simulink model "vector"  (R2025a)
settings: Solver=VariableStepAuto  StartTime=0.0  StopTime=5  RelTol=1e-3
libraries: spsCurrentMeasurementLib x3, spsVoltageMeasurementLib x2, spsAsynchronousMachineSIUnitsLib x1, spsDCVoltageSourceLib x1, eeHysteresisControl x1, spsUniversalBridgeLib x1, sps_lib x1
settings Model: Creator=aditl  LastModifiedBy=aditl

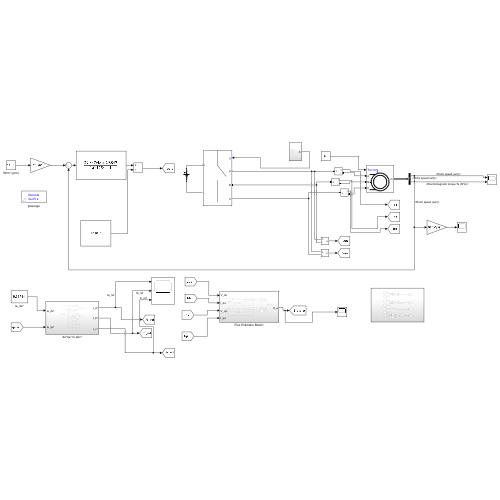
[thumbnail: Simulink's stored preview of the top-level diagram]
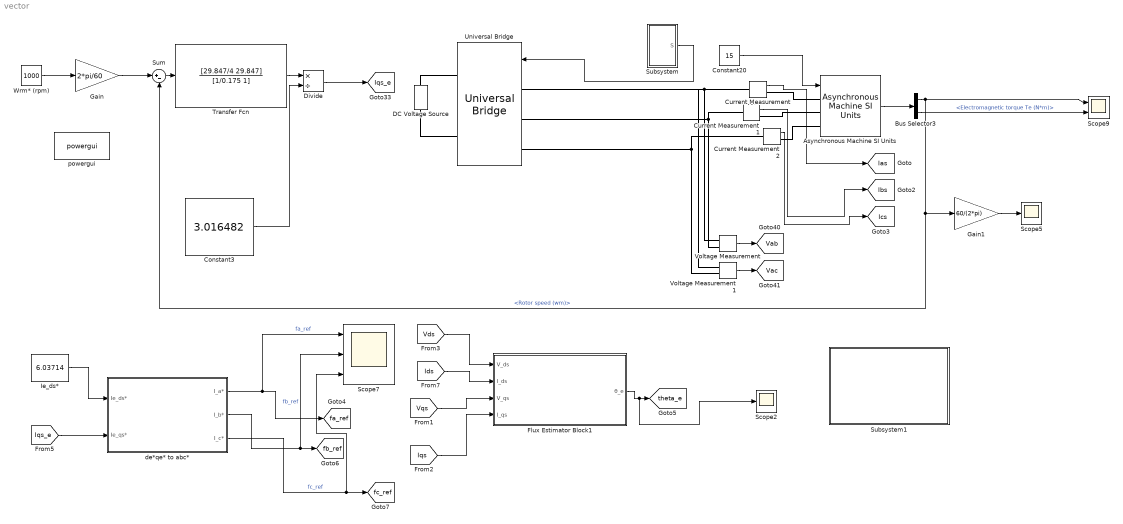
== system vector ==
  Asynchronous Machine SI Units : spsAsynchronousMachineSIUnitsLib/Asynchronous Machine SI Units  RotorType=Squirrel-cage  PresetModel="15:  5.4 HP (4KW)   400 V  50Hz 1430 RPM"  MechanicalLoad=Torque Tm  ShowDetailedParameters=on  ReferenceFrame=Stationary  Units=SI  MeasurementBus=off  NominalParameters=[4000 400 50]  VoltageRatio=1  Stator=[1.405 0.005839]  Rotor=[1.395 0.005839]  Cage1=[0.4155 0.002066]  Cage2=[0.4168 0.0003495]  Lm=0.1722  Mechanical=[0.0131 0.002985 2]  PolePairs=2  InitialConditions=[0 10 0 0 0 0 0 0]  SimulateSaturation=off  Saturation=[14.03593122, 27.81365428, 53.79336849, 72.68890987, 97.98006896, 148.6815601, 215.7428561, 302.9841135, 428.7778367 ; 230, 322, 414, 460, 506, 552, 598, 644, 690]  LoadFlowParameters=1492000  TsPowergui=0  TsBlock=-1  IterativeModel=Trapezoidal non iterative  IterativeDiscreteModel=Trapezoidal non iterative  Pmec=1.492e+006
  Bus Selector3 : BusSelector  OutputSignals=Mechanical.Rotor speed (wm),Mechanical.Electromagnetic torque Te (N*m)
  Constant20 : Constant  Value=15
  Constant3 : Constant  Value=3.016482
  Current Measurement : spsCurrentMeasurementLib/Current Measurement  PhasorSimulation=off  OutputType=Complex  PSBequivalent=0
  Current Measurement1 : spsCurrentMeasurementLib/Current Measurement  PhasorSimulation=off  OutputType=Complex  PSBequivalent=0
  Current Measurement2 : spsCurrentMeasurementLib/Current Measurement  PhasorSimulation=off  OutputType=Complex  PSBequivalent=0
  DC Voltage Source : spsDCVoltageSourceLib/DC Voltage Source  Amplitude=1088.662  Measurements=None
  Divide : Product  Inputs=*/
  Flux Estimator Block1 : Subsystem
  Gain : Gain  Gain=2*pi/60
  Gain1 : Gain  Gain=60/(2*pi)
  Ie_ds* : Constant  Value=6.03714
  Scope2 : Scope
      settings: ActiveDisplayYMinimum=-3.926985235827948  ActiveDisplayYMaximum=3.9269805856564539
  Scope5 : Scope
      settings: ActiveDisplayYMinimum=-1164.848987364373  ActiveDisplayYMaximum=1796.0943319293749  DataLoggingVariableName=ScopeData5
  Scope7 : Scope  NumInputPorts=3
      settings: ActiveDisplayYMinimum=-753403.64622958587  ActiveDisplayYMaximum=359759.36964912462  DataLoggingVariableName=ScopeData7
  Scope9 : Scope  NumInputPorts=2
      settings: ActiveDisplayYMinimum=45.4669289684437  ActiveDisplayYMaximum=169.48104420293922  DataLoggingVariableName=ScopeData9
  Subsystem : Subsystem
  Subsystem1 : Subsystem
  Sum : Sum  Inputs=|+-
  Transfer Fcn : TransferFcn  Numerator=[29.847/4 29.847]  Denominator=[1/0.175 1]
  Universal Bridge : spsUniversalBridgeLib/Universal Bridge  Arms=3  SnubberResistance=1e5  SnubberCapacitance=inf  Device=Ideal Switches  Ron=1e-3  Lon=0  ForwardVoltages="[  0  0  ]"  ForwardVoltage=0  GTOparameters=[ 10e-6 , 20e-6 ]  IGBTparameters=[ 1e-6 , 2e-6 ]  Measurements=None  Measurements_2=None  converterType=Rectifier
  Voltage Measurement : spsVoltageMeasurementLib/Voltage Measurement  PhasorSimulation=off  OutputType=Complex  PSBequivalent=0
  Voltage Measurement1 : spsVoltageMeasurementLib/Voltage Measurement  PhasorSimulation=off  OutputType=Complex  PSBequivalent=0
  Wrm* (rpm) : Constant  Value=1000
  de*qe* to abc* : Subsystem
  powergui : sps_lib/powergui  Priority=1  SimulationMode=Discrete  SampleTime=50e-6  frequency=60  Iterations=50  frequencyindice=50  Pbase=100e6  ErrMax=1e-4  UnitsV=kV  UnitsW=MW  buscounter=0  FunctionMessages=off  echomessages=off  EnableUseOfTLC=off  CurrentSourceSwitches=off  DisableSnubberDevices=off  DisableRonSwitches=off  DisableVfSwitches=off  DisplayEquations=off  AutomaticDiscreteSolvers=off  SolverType=Tustin/Backward Euler (TBE)  Interpol=off  ExternalGateDelay=off  methode=off  Ts=100  x0status=blocks  SPID=on  SwTol=0  HookPort=off  NonlinearTolerance=1e-4  nMaxIteration=100  ContinueOnMaxIteration=off  RestoreLinks=warning  ResistiveCurrentMeasurement=off  Frange=[0:2:500]  Ylog=off  Xlog=on  ShowGrid=off  save=off  variable=ZData  structure=0  ZoomFFT=off  StartTime=0.0  cycles=1  DisplayStyle=1  fundamental=60  FreqAxis=off  MaxFrequency=1000  frequencyindicesteady=1  RmsSteady=1  display=off
  tag scope: Ias=global, Ibs=global, Ics=global, Iqs_e=global, Vab=global, Vac=global, fa_ref=global, fb_ref=global, fc_ref=global, theta_e=global
  wires:
  de*qe* to abc*/2(I_b*) -> Scope7/2, [fb_ref]  "fb_ref"
  Wrm* (rpm)/1 -> Gain/1
  Bus Selector3/1 -> Gain1/1, Sum/2, Scope9/1  "<Rotor speed (wm)>"
  Transfer Fcn/1 -> Divide/1
  Gain/1 -> Sum/1
  Current Measurement/1 -> [Ias]
  de*qe* to abc*/1(I_a*) -> Scope7/1, [fa_ref]  "fa_ref"
  Sum/1 -> Transfer Fcn/1
  Current Measurement2/1 -> [Ics]
  Bus Selector3/2 -> Scope9/2  "<Electromagnetic torque Te (N*m)>"
  de*qe* to abc*/3(I_c*) -> Scope7/3, [fc_ref]  "fc_ref"
  Divide/1 -> [Iqs_e]
  Voltage Measurement/1 -> [Vab]
  Gain1/1 -> Scope5/1
  Asynchronous Machine SI Units/1 -> Bus Selector3/1
  Current Measurement1/1 -> [Ibs]
  Voltage Measurement1/1 -> [Vac]
  Constant20/1 -> Asynchronous Machine SI Units/1
  [Iqs_e] -> de*qe* to abc*/2(Ie_qs*)
  Constant3/1 -> Divide/2
  Ie_ds*/1 -> de*qe* to abc*/1(Ie_ds*)
  Subsystem/1(S) -> Universal Bridge/1
  Flux Estimator Block1/1(θ_e) -> [theta_e], Scope2/1
  [Iqs] -> Flux Estimator Block1/4(I_qs)
  [Vqs] -> Flux Estimator Block1/3(V_qs)
  [Ids] -> Flux Estimator Block1/2(I_ds)
  [Vds] -> Flux Estimator Block1/1(V_ds)
  connections:
  Voltage Measurement/LConn1 -- Universal Bridge/LConn1 -- Voltage Measurement1/LConn1 -- Current Measurement/LConn1
  Voltage Measurement/LConn2 -- Current Measurement1/LConn1 -- Universal Bridge/LConn2
  Voltage Measurement1/LConn2 -- Current Measurement2/LConn1 -- Universal Bridge/LConn3
  Current Measurement/RConn1 -- Asynchronous Machine SI Units/LConn1
  Current Measurement2/RConn1 -- Asynchronous Machine SI Units/LConn3
  Current Measurement1/RConn1 -- Asynchronous Machine SI Units/LConn2
  DC Voltage Source/RConn1 -- Universal Bridge/RConn1
  DC Voltage Source/LConn1 -- Universal Bridge/RConn2

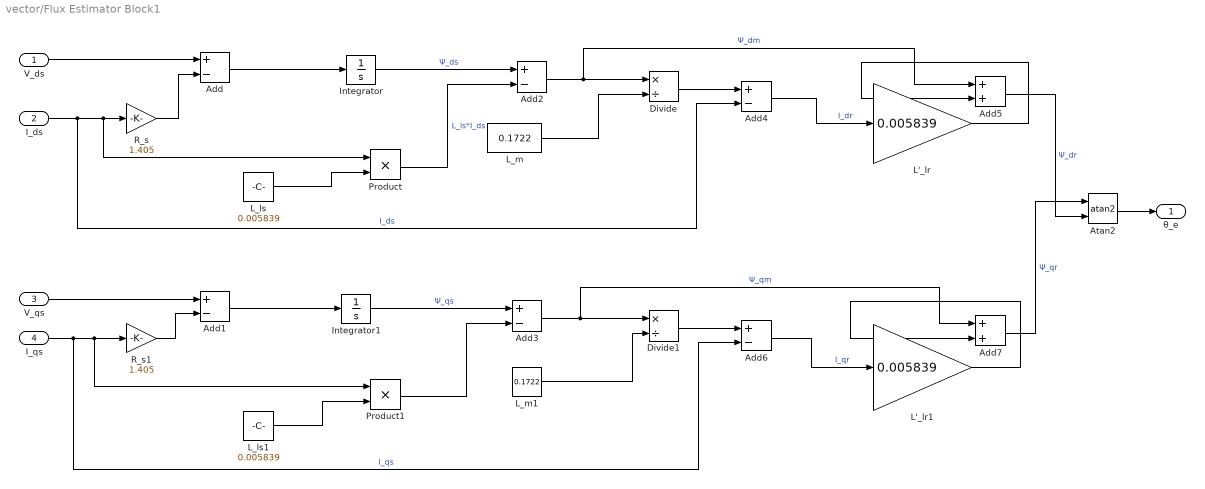
== system vector/Flux Estimator Block1 ==
  V_ds : Inport
  I_ds : Inport  Port=2
  V_qs : Inport  Port=3
  I_qs : Inport  Port=4
  Add{,1..4,6} (6 alike) : Sum  Inputs=+-
  Add5 : Sum
  Add7 : Sum
  Atan2 : Trigonometry  Operator=atan2
  Divide : Product  Inputs=*/
  Divide1 : Product  Inputs=*/
  Integrator : Integrator
  Integrator1 : Integrator
  L'_lr : Gain  Gain=0.005839
  L'_lr1 : Gain  Gain=0.005839
  L_ls : Constant  Value=0.005839
  L_ls1 : Constant  Value=0.005839
  L_m : Constant  Value=0.1722
  L_m1 : Constant  Value=0.1722
  Product : Product
  Product1 : Product
  R_s : Gain  Gain=1.405
  R_s1 : Gain  Gain=1.405
  θ_e : Outport
  wires:
  Atan2/1 -> θ_e/1
  Divide1/1 -> Add6/1
  Add6/1 -> L'_lr1/1  "I_qr"
  L'_lr1/1 -> Add7/2
  Add7/1 -> Atan2/1  "Ψ_qr"
  Add5/1 -> Atan2/2  "Ψ_dr"
  L'_lr/1 -> Add5/2
  Add4/1 -> L'_lr/1  "I_dr"
  Divide/1 -> Add4/1
  L_m1/1 -> Divide1/2
  Add3/1 -> Divide1/1, Add7/1  "Ψ_qm"
  L_m/1 -> Divide/2
  Add2/1 -> Divide/1, Add5/1  "Ψ_dm"
  Product1/1 -> Add3/2
  L_ls1/1 -> Product1/2
  Product/1 -> Add2/2  "L_ls*I_ds"
  L_ls/1 -> Product/2
  Integrator1/1 -> Add3/1  "Ψ_qs"
  Integrator/1 -> Add2/1  "Ψ_ds"
  Add1/1 -> Integrator1/1
  Add/1 -> Integrator/1
  V_qs/1 -> Add1/1
  R_s1/1 -> Add1/2
  V_ds/1 -> Add/1
  R_s/1 -> Add/2
  I_ds/1 -> R_s/1, Product/1, Add4/2  "I_ds"
  I_qs/1 -> Product1/1, R_s1/1, Add6/2  "I_qs"

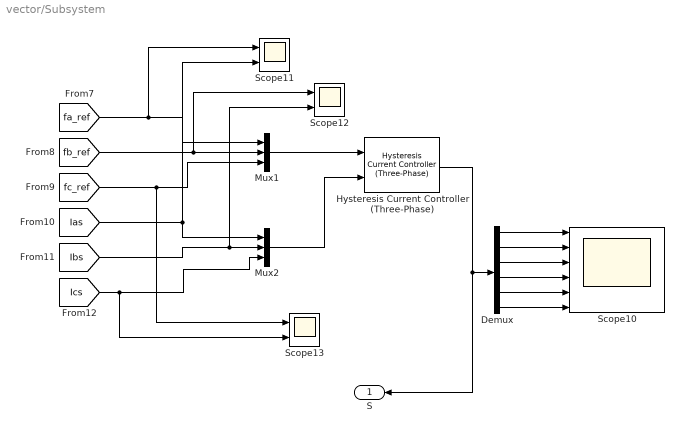
== system vector/Subsystem ==
  Demux : Demux  Outputs=6
  Hysteresis Current Controller (Three-Phase) : eeHysteresisControl/Hysteresis Current Controller (Three-Phase)  h=1.3  Ts=-1
      settings: LibrarySourceBlock=|
      | ee_sl_lib/General Machine
      | Control/Hysteresis Current
      | Controller
      | (Three-Phase)
  Mux1 : Mux  Inputs=3
  Mux2 : Mux  Inputs=3
  Scope10 : Scope  NumInputPorts=6
      settings: ActiveDisplayYMinimum=-0.12499999999999997  ActiveDisplayYMaximum=1.125  DataLoggingVariableName=ScopeData11
  Scope11 : Scope  NumInputPorts=2
      settings: ActiveDisplayYMinimum=1.6721282372561657  ActiveDisplayYMaximum=63.451918813451442  DataLoggingVariableName=ScopeData12
  Scope12 : Scope  NumInputPorts=2
      settings: ActiveDisplayYMinimum=-78.434145790718887  ActiveDisplayYMaximum=2.5704136454950897  DataLoggingVariableName=ScopeData13
  Scope13 : Scope  NumInputPorts=2
      settings: ActiveDisplayYMinimum=-68.536634079904516  ActiveDisplayYMaximum=41.352885154542406  DataLoggingVariableName=ScopeData14
  S : Outport
  wires:
  Hysteresis Current Controller (Three-Phase)/1 -> S/1, Demux/1
  [Ias] -> Scope11/2, Mux2/1
  Demux/5 -> Scope10/5
  [Ics] -> Scope13/2, Mux2/3
  [Ibs] -> Scope12/2, Mux2/2
  Demux/4 -> Scope10/4
  Mux1/1 -> Hysteresis Current Controller (Three-Phase)/1
  [fa_ref] -> Scope11/1, Mux1/1
  Demux/1 -> Scope10/1
  [fc_ref] -> Scope13/1, Mux1/3
  [fb_ref] -> Scope12/1, Mux1/2
  Mux2/1 -> Hysteresis Current Controller (Three-Phase)/2
  Demux/3 -> Scope10/3
  Demux/2 -> Scope10/2
  Demux/6 -> Scope10/6

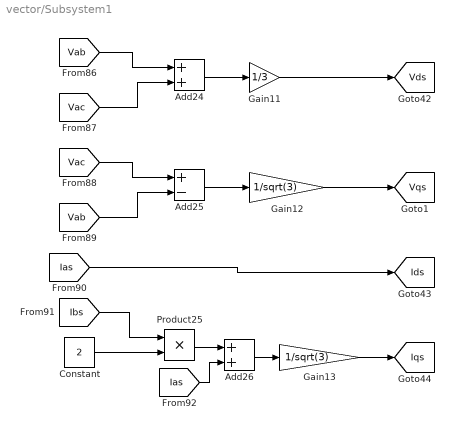
== system vector/Subsystem1 ==
  Add24 : Sum
  Add25 : Sum  Inputs=+-
  Add26 : Sum
  Constant : Constant  Value=2
  Gain11 : Gain  Gain=1/3
  Gain12 : Gain  Gain=1/sqrt(3)
  Gain13 : Gain  Gain=1/sqrt(3)
  Product25 : Product
  tag scope: Ids=global, Iqs=global, Vds=global, Vqs=global
  wires:
  [Vac] -> Add24/2
  Gain12/1 -> [Vqs]
  Add25/1 -> Gain12/1
  Gain13/1 -> [Iqs]
  [Vab] -> Add25/2
  Constant/1 -> Product25/2
  [Ias] -> Add26/2
  Add24/1 -> Gain11/1
  [Vab] -> Add24/1
  Product25/1 -> Add26/1
  [Ias] -> [Ids]
  [Vac] -> Add25/1
  Add26/1 -> Gain13/1
  [Ibs] -> Product25/1
  Gain11/1 -> [Vds]

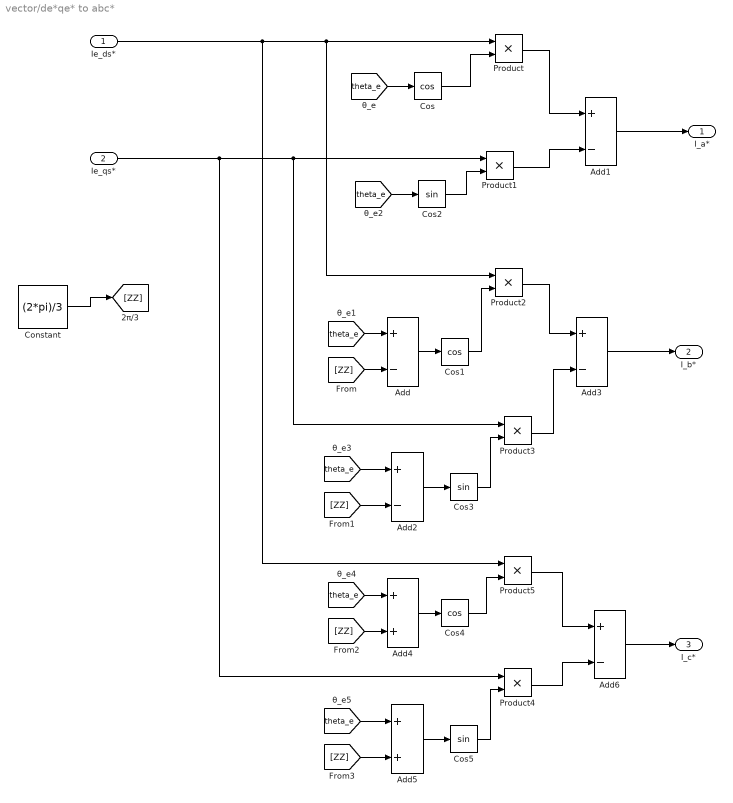
== system vector/de*qe* to abc* ==
  Ie_ds* : Inport
  Ie_qs* : Inport  Port=2
  Add{,1..3,6} (5 alike) : Sum  Inputs=+-
  Add4 : Sum
  Add5 : Sum
  Constant : Constant  Value=(2*pi)/3
  Cos : Trigonometry  Operator=cos
  Cos1 : Trigonometry  Operator=cos
  Cos2 : Trigonometry
  Cos3 : Trigonometry
  Cos4 : Trigonometry  Operator=cos
  Cos5 : Trigonometry
  Product{,1..5} (6 alike) : Product
  I_a* : Outport
  I_b* : Outport  Port=2
  I_c* : Outport  Port=3
  wires:
  Constant/1 -> [ZZ]
  [theta_e] -> Cos/1
  Add/1 -> Cos1/1
  Ie_ds*/1 -> Product5/1, Product2/1, Product/1
  Cos/1 -> Product/2
  Cos2/1 -> Product1/2
  [theta_e] -> Cos2/1
  Ie_qs*/1 -> Product4/1, Product3/1, Product1/1
  Product1/1 -> Add1/2
  Product/1 -> Add1/1
  Add1/1 -> I_a*/1
  Add2/1 -> Cos3/1
  [ZZ] -> Add/2
  [theta_e] -> Add/1
  [ZZ] -> Add2/2
  [theta_e] -> Add2/1
  Cos1/1 -> Product2/2
  Cos3/1 -> Product3/2
  Product2/1 -> Add3/1
  Product3/1 -> Add3/2
  [theta_e] -> Add4/1
  [ZZ] -> Add4/2
  Add4/1 -> Cos4/1
  Cos5/1 -> Product4/2
  [theta_e] -> Add5/1
  [ZZ] -> Add5/2
  Add5/1 -> Cos5/1
  Product4/1 -> Add6/2
  Cos4/1 -> Product5/2
  Add3/1 -> I_b*/1
  Add6/1 -> I_c*/1
  Product5/1 -> Add6/1
